simulink model "sustem4"  (R2018b)
settings: Solver=VariableStepAuto  StartTime=0.0  StopTime=10.0  RelTol=1e-3
libraries: cstblocks x2
settings Model: Creator=Abraham Pérez  LastModifiedBy=Abraham Pérez

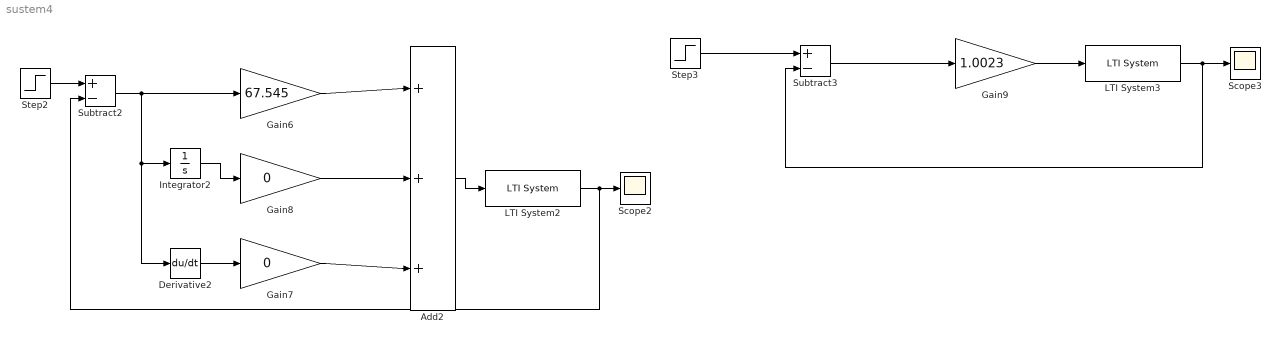
== system sustem4 ==
  Add2 : Sum  Inputs=+++
  Derivative2 : Derivative
  Gain6 : Gain  Gain=67.545
  Gain7 : Gain  Gain=0
  Gain8 : Gain  Gain=0
  Gain9 : Gain  Gain=1.0023
  Integrator2 : Integrator
  LTI System2 : cstblocks/LTI System  sys=G4  IC=[]
  LTI System3 : cstblocks/LTI System  sys=G4  IC=[]
  Scope2 : Scope
  Scope3 : Scope
  Step2 : Step  Time=0  After=9  SampleTime=0
  Step3 : Step  Time=0  SampleTime=0
  Subtract2 : Sum  Inputs=+-
  Subtract3 : Sum  Inputs=+-
  wires:
  LTI System3/1 -> Subtract3/2, Scope3/1
  LTI System2/1 -> Subtract2/2, Scope2/1
  Step3/1 -> Subtract3/1
  Subtract2/1 -> Derivative2/1, Integrator2/1, Gain6/1
  Gain9/1 -> LTI System3/1
  Integrator2/1 -> Gain8/1
  Add2/1 -> LTI System2/1
  Gain8/1 -> Add2/2
  Step2/1 -> Subtract2/1
  Gain6/1 -> Add2/1
  Subtract3/1 -> Gain9/1
  Derivative2/1 -> Gain7/1
  Gain7/1 -> Add2/3
